simulink model "InvDynControl"  (Simulink 7.9)
settings: Solver=ode45  StartTime=0.0  StopTime=10.0  RelTol=1e-3
undefined symbols (not defined in the file): kd1, kd2, kd3, kd4, kd5, kd6, kp1, kp2, kp3, kp4, kp5, kp6, LinePTs2Rpm, PosSourceSelect, Ts
libraries: powerlib_extras x3
settings Model: Creator=Administrator  LastModifiedBy=Administrator

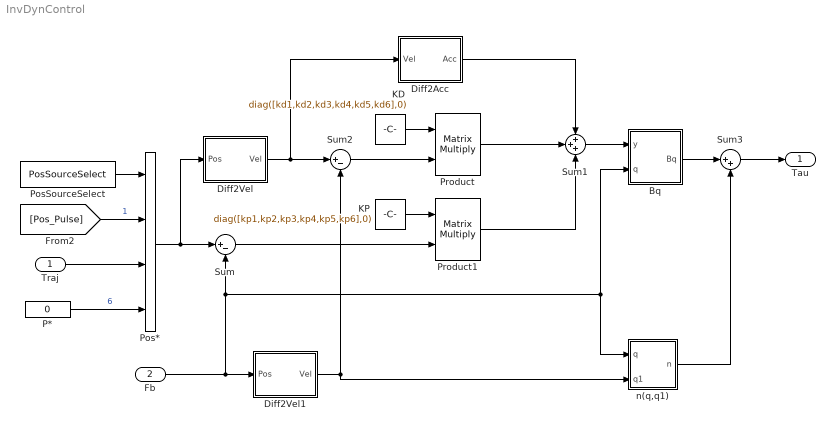
== system InvDynControl ==
  Traj : Inport
  Fb : Inport  Port=2
  Bq : Subsystem
  Diff2Acc : Subsystem
  Diff2Vel : Subsystem
  Diff2Vel1 : Subsystem
  KD : Constant  Value=diag([kd1,kd2,kd3,kd4,kd5,kd6],0)
  KP : Constant  Value=diag([kp1,kp2,kp3,kp4,kp5,kp6],0)
  P* : Constant  Value=0  SampleTime=Ts
  Pos* : MultiPortSwitch  zeroidx=off  SampleTime=Ts
  PosSourceSelect : Constant  Value=PosSourceSelect  SampleTime=Ts
  Product : Product  Multiplication=Matrix(*)  RndMeth=Zero
  Product1 : Product  Multiplication=Matrix(*)  RndMeth=Zero
  Sum : Sum  Inputs=|+-  SampleTime=Ts
  Sum1 : Sum  Inputs=+++  SampleTime=Ts
  Sum2 : Sum  Inputs=|+-  SampleTime=Ts
  Sum3 : Sum  Inputs=|++  SampleTime=Ts
  n(q,q1) : Subsystem
  Tau : Outport
  wires:
  [Pos_Pulse] -> Pos*/2  "1"
  P*/1 -> Pos*/4  "6"
  PosSourceSelect/1 -> Pos*/1
  Diff2Vel/1(Vel) -> Sum2/1, Diff2Acc/1(Vel)
  Diff2Acc/1(Acc) -> Sum1/1
  Diff2Vel1/1(Vel) -> Sum2/2, n(q,q1)/2(q1)
  Sum1/1 -> Bq/1(y)
  Bq/1(Bq) -> Sum3/1
  n(q,q1)/1(n) -> Sum3/2
  Sum3/1 -> Tau/1
  Traj/1 -> Pos*/3
  Product/1 -> Sum1/2
  Sum/1 -> Product1/2
  Product1/1 -> Sum1/3
  Sum2/1 -> Product/2
  KD/1 -> Product/1
  KP/1 -> Product1/1
  Pos*/1 -> Sum/1, Diff2Vel/1(Pos)
  Fb/1 -> Diff2Vel1/1(Pos), Sum/2, Bq/2(q), n(q,q1)/1(q)

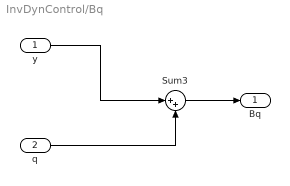
== system InvDynControl/Bq ==
  y : Inport
  q : Inport  Port=2
  Sum3 : Sum  Inputs=|++
  Bq : Outport
  wires:
  q/1 -> Sum3/2
  y/1 -> Sum3/1
  Sum3/1 -> Bq/1

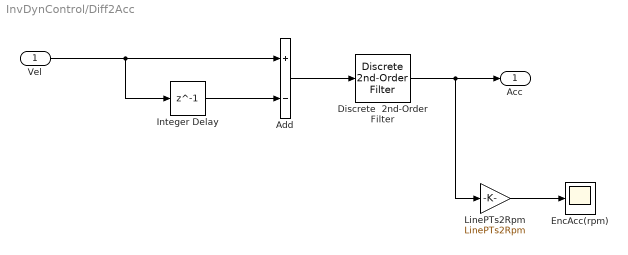
== system InvDynControl/Diff2Acc ==
  Vel : Inport
  Add : Sum  Inputs=+-
  Discrete  2nd-Order Filter : powerlib_extras/Discrete  Control Blocks/Discrete  2nd-Order Filter  FilterType=Lowpass  Fo=200  Zeta=0.707  Ts=Ts  Initialize=off  Vac_Init=[0.8 -25 60]  Vdc_Init=-0.4  PlotResponse=off  param1=[1 5000 10]
  EncAcc(rpm) : Scope
      settings: SaveName=ScopeData33
  Integer Delay : Delay  DelayLength=1  InputProcessing=Inherited
  LinePTs2Rpm : Gain  Gain=LinePTs2Rpm
  Acc : Outport
  wires:
  Add/1 -> Discrete  2nd-Order Filter/1
  Discrete  2nd-Order Filter/1 -> Acc/1, LinePTs2Rpm/1
  Vel/1 -> Integer Delay/1, Add/1
  Integer Delay/1 -> Add/2
  LinePTs2Rpm/1 -> EncAcc(rpm)/1

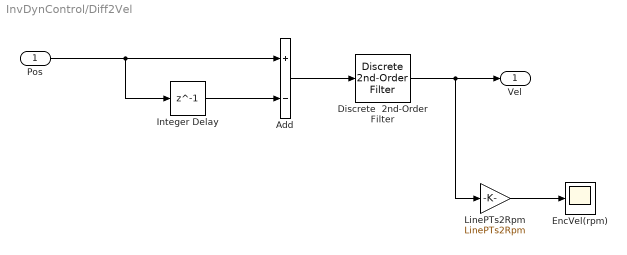
== system InvDynControl/Diff2Vel ==
  Pos : Inport
  Add : Sum  Inputs=+-
  Discrete  2nd-Order Filter : powerlib_extras/Discrete  Control Blocks/Discrete  2nd-Order Filter  FilterType=Lowpass  Fo=200  Zeta=0.707  Ts=Ts  Initialize=off  Vac_Init=[0.8 -25 60]  Vdc_Init=-0.4  PlotResponse=off  param1=[1 5000 10]
  EncVel(rpm) : Scope
      settings: SaveName=ScopeData33
  Integer Delay : Delay  DelayLength=1  InputProcessing=Inherited
  LinePTs2Rpm : Gain  Gain=LinePTs2Rpm
  Vel : Outport
  wires:
  Add/1 -> Discrete  2nd-Order Filter/1
  Discrete  2nd-Order Filter/1 -> Vel/1, LinePTs2Rpm/1
  Pos/1 -> Integer Delay/1, Add/1
  Integer Delay/1 -> Add/2
  LinePTs2Rpm/1 -> EncVel(rpm)/1

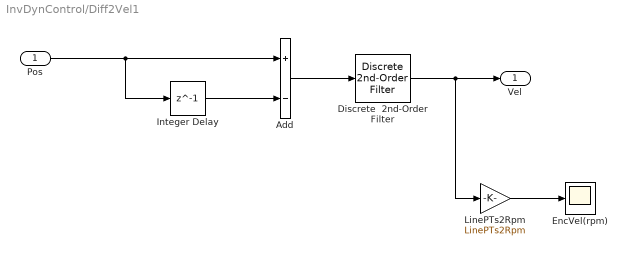
== system InvDynControl/Diff2Vel1 ==
  Pos : Inport
  Add : Sum  Inputs=+-
  Discrete  2nd-Order Filter : powerlib_extras/Discrete  Control Blocks/Discrete  2nd-Order Filter  FilterType=Lowpass  Fo=200  Zeta=0.707  Ts=Ts  Initialize=off  Vac_Init=[0.8 -25 60]  Vdc_Init=-0.4  PlotResponse=off  param1=[1 5000 10]
  EncVel(rpm) : Scope
      settings: SaveName=ScopeData33
  Integer Delay : Delay  DelayLength=1  InputProcessing=Inherited
  LinePTs2Rpm : Gain  Gain=LinePTs2Rpm
  Vel : Outport
  wires:
  Add/1 -> Discrete  2nd-Order Filter/1
  Discrete  2nd-Order Filter/1 -> Vel/1, LinePTs2Rpm/1
  Pos/1 -> Integer Delay/1, Add/1
  Integer Delay/1 -> Add/2
  LinePTs2Rpm/1 -> EncVel(rpm)/1

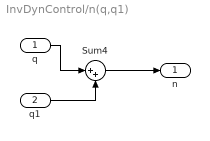
== system InvDynControl/n(q,q1) ==
  q : Inport
  q1 : Inport  Port=2
  Sum4 : Sum  Inputs=|++  SampleTime=Ts
  n : Outport
  wires:
  Sum4/1 -> n/1
  q/1 -> Sum4/1
  q1/1 -> Sum4/2
